simulink model "Linear_Moving_Setpoint_SS_Int"  (R2021b)
settings: Solver=VariableStepAuto  StartTime=tspan(1)  StopTime=tspan(2)  RelTol=1e-9
undefined symbols (not defined in the file): K1, K2, r_sim, x_0
settings Model: Creator=domin  LastModifiedBy=domin
settings SolverCC: AlgebraicLoopSolver=TrustRegion
settings DebuggingCC: SFMachineParentedDataDiag=warning

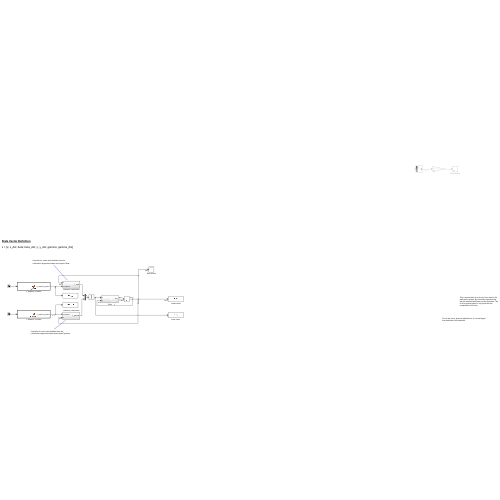
[thumbnail: Simulink's stored preview of the top-level diagram]
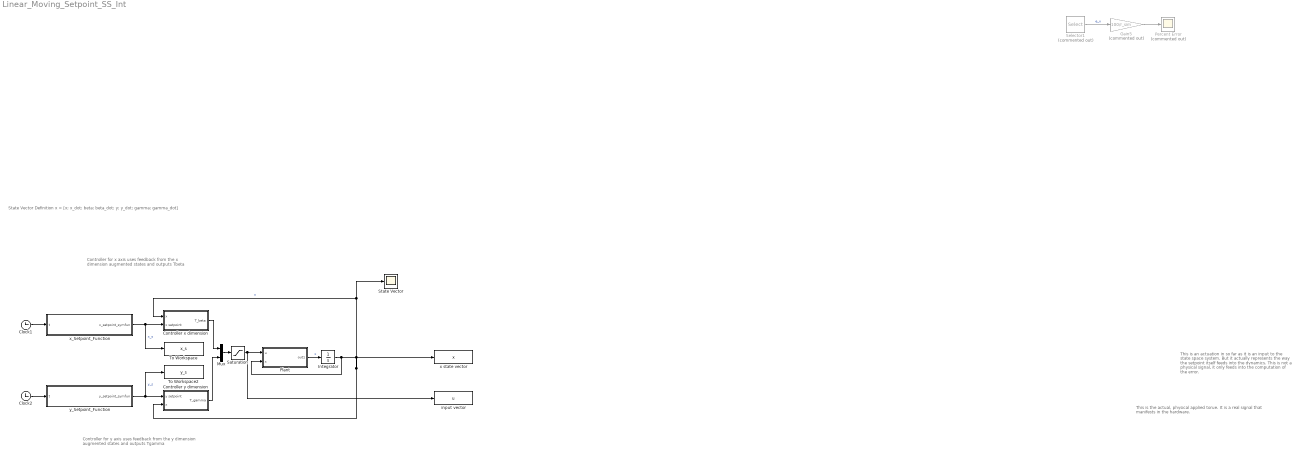
== system Linear_Moving_Setpoint_SS_Int ==
  note: Controller for y axis uses feedback from the
      | y dimension augmented states and outputs Tgamma
  note: State Vector Definition
      |
      | x = [x; x_dot; beta; beta_dot; y; y_dot; gamma; gamma_dot]
  note: This is the actual, physical applied torue. It is a real signal
      | that manifests in the hardware.
  note: This is an actuation in so far as it is an input to the
      | state space system. But it actually represents the
      | way the setpoint itself feeds into the dynamics. This
      | is not a physical signal, it only feeds into the
      | computation of the error.
  note: Controller for x axis uses feedback from the
      | x dimension augmented states and outputs Tbeta
  Clock1 : Clock
  Clock2 : Clock
  Controller x dimension : Subsystem
  Controller y dimension : Subsystem
  Gain5 : Gain  Commented=on  Gain=100/r_sim
  Integrator : Integrator  InitialCondition=x_0
  Mux : Mux  Inputs=2
  Percent Error : Scope  Commented=on
  Plant : Subsystem
  Saturation : Saturate  UpperLimit=73/1000  LowerLimit=-73/1000
  Selector1 : Selector  Commented=on  InputPortWidth=5  IndexOptions=Index vector (dialog)  Indices=[1]  OutputSizes=1
  State Vector : Scope
  To Workspace : ToWorkspace  VariableName=x_s  SampleTime=-1
  To Workspace2 : ToWorkspace  VariableName=y_s  SampleTime=-1
  input vector : ToWorkspace  VariableName=u  SampleTime=-1
  x state vector : ToWorkspace  VariableName=x  SampleTime=-1
  x_Setpoint_Function : MATLAB Function  TreatAsAtomicUnit=on
  y_Setpoint_Function : MATLAB Function  TreatAsAtomicUnit=on
  wires:
  Integrator/1 -> Plant/2(x), x state vector/1, Controller x dimension/1(x), State Vector/1, Controller y dimension/2(x)  "x"
  Plant/1(out1) -> Integrator/1  "x"
  Clock1/1 -> x_Setpoint_Function/1(t)
  Gain5/1 -> Percent Error/1
  Selector1/1 -> Gain5/1  "e_x"
  Clock2/1 -> y_Setpoint_Function/1(t)
  Controller x dimension/1(T_beta) -> Mux/1
  Controller y dimension/1(T_gamma) -> Mux/2
  x_Setpoint_Function/1(x_setpoint_symfun) -> To Workspace/1, Controller x dimension/2(x setpoint)  "x_s"
  y_Setpoint_Function/1(y_setpoint_symfun) -> To Workspace2/1, Controller y dimension/1(y setpoint)  "y_s"
  Mux/1 -> Saturation/1
  Saturation/1 -> Plant/1(u), input vector/1

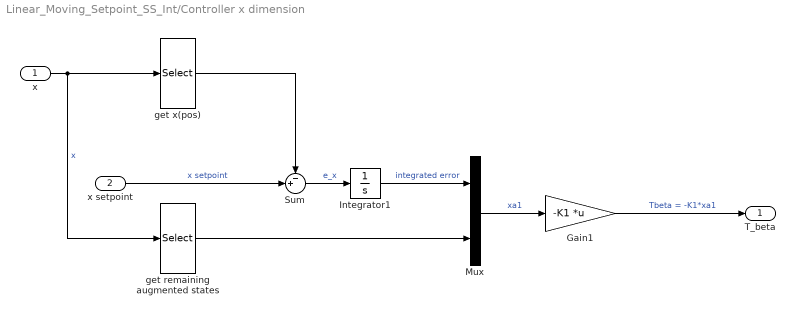
== system Linear_Moving_Setpoint_SS_Int/Controller x dimension ==
  x : Inport
  x setpoint : Inport  Port=2
  Gain1 : Gain  Gain=-K1  Multiplication=Matrix(K*u)
  Integrator1 : Integrator
  Mux : Mux  Inputs=2
  Sum : Sum  Inputs=-+|
  get remaining augmented states : Selector  InputPortWidth=8  IndexOptions=Index vector (dialog)  Indices=[1,2,3,4]  OutputSizes=1
  get x(pos) : Selector  InputPortWidth=8  IndexOptions=Index vector (dialog)  Indices=[1]  OutputSizes=1
  T_beta : Outport
  wires:
  get remaining augmented states/1 -> Mux/2
  Gain1/1 -> T_beta/1  "Tbeta = -K1*xa1"
  get x(pos)/1 -> Sum/1
  Mux/1 -> Gain1/1  "xa1"
  Sum/1 -> Integrator1/1  "e_x"
  Integrator1/1 -> Mux/1  "integrated error"
  x setpoint/1 -> Sum/2  "x setpoint"
  x/1 -> get remaining augmented states/1, get x(pos)/1  "x"

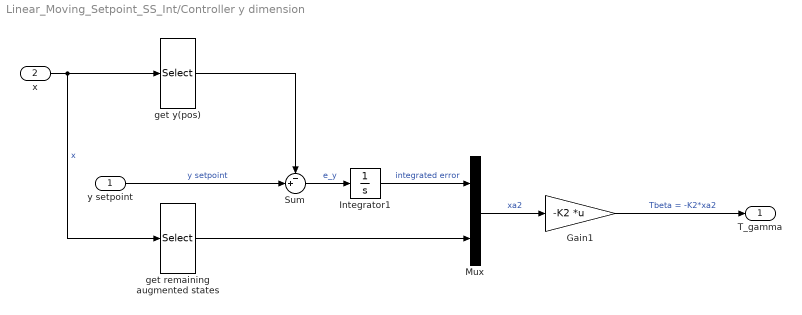
== system Linear_Moving_Setpoint_SS_Int/Controller y dimension ==
  y setpoint : Inport
  x : Inport  Port=2
  Gain1 : Gain  Gain=-K2  Multiplication=Matrix(K*u)
  Integrator1 : Integrator
  Mux : Mux  Inputs=2
  Sum : Sum  Inputs=-+|
  get remaining augmented states : Selector  InputPortWidth=8  IndexOptions=Index vector (dialog)  Indices=[5,6,7,8]  OutputSizes=1
  get y(pos) : Selector  InputPortWidth=8  IndexOptions=Index vector (dialog)  Indices=[2]  OutputSizes=1
  T_gamma : Outport
  wires:
  x/1 -> get y(pos)/1, get remaining augmented states/1  "x"
  y setpoint/1 -> Sum/2  "y setpoint"
  Integrator1/1 -> Mux/1  "integrated error"
  Sum/1 -> Integrator1/1  "e_y"
  Mux/1 -> Gain1/1  "xa2"
  get y(pos)/1 -> Sum/1
  Gain1/1 -> T_gamma/1  "Tbeta = -K2*xa2"
  get remaining augmented states/1 -> Mux/2

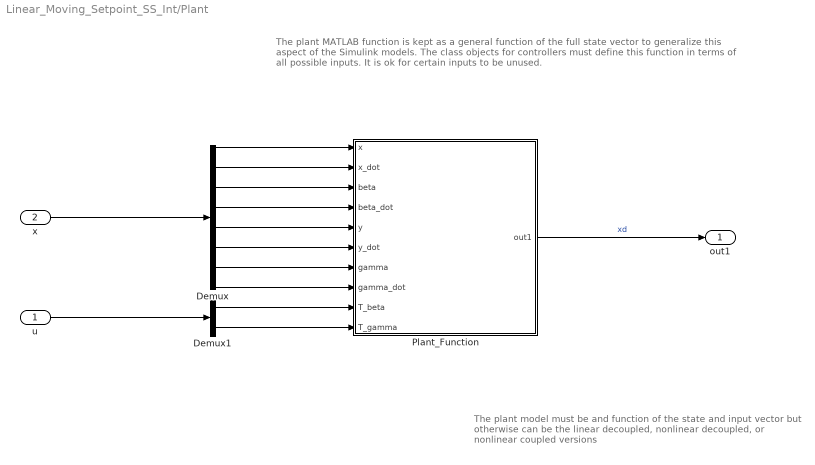
== system Linear_Moving_Setpoint_SS_Int/Plant ==
  note: The plant model must be and function of the state and input vector
      |  but otherwise can be the linear decoupled, nonlinear decoupled,
      | or nonlinear coupled versions
  note: The plant MATLAB function is kept as a general function of the full state vector
      | to generalize this aspect of the Simulink models. The class objects for controllers must define this function in terms of all possible inputs. It is ok for certain inputs to be unused.
  u : Inport
  x : Inport  Port=2
  Demux : Demux  Outputs=8
  Demux1 : Demux  Outputs=2
  Plant_Function : MATLAB Function  TreatAsAtomicUnit=on
  out1 : Outport
  wires:
  Demux/1 -> Plant_Function/1(x)
  x/1 -> Demux/1
  Plant_Function/1(out1) -> out1/1  "xd"
  Demux/2 -> Plant_Function/2(x_dot)
  Demux/4 -> Plant_Function/4(beta_dot)
  Demux/3 -> Plant_Function/3(beta)
  Demux/6 -> Plant_Function/6(y_dot)
  Demux/5 -> Plant_Function/5(y)
  Demux1/2 -> Plant_Function/10(T_gamma)
  u/1 -> Demux1/1
  Demux/8 -> Plant_Function/8(gamma_dot)
  Demux1/1 -> Plant_Function/9(T_beta)
  Demux/7 -> Plant_Function/7(gamma)

== matlab function Linear_Moving_Setpoint_SS_Int/Plant/Plant_Function ==
  data: x input; out1 output; x_dot input; beta input; beta_dot input; y input; y_dot input; gamma input; gamma_dot input; T_beta input; T_gamma input
function out1 = xdot(x,x_dot,beta,beta_dot,y,y_dot,gamma,gamma_dot,T_beta,T_gamma)
%#codegen

%    This function was generated by the Symbolic Math Toolbox version 9.0.
%    04-Nov-2021 01:00:01

mt1 = [x_dot,T_beta.*(-1.772680446266138e+1)+beta.*4.011095116498257-x.*5.216998553361243,beta_dot,T_beta.*3.835784582337856e+2+beta.*6.482947197685378e+1+x.*1.128871402582031e+2,y_dot,T_gamma.*1.772680446266138e+1-gamma.*4.011095116498257-y.*5.216998553361243,gamma_dot];
mt2 = [T_gamma.*3.835784582337856e+2+gamma.*6.482947197685378e+1-y.*1.128871402582031e+2];
out1 = reshape([mt1,mt2],8,1);

== matlab function Linear_Moving_Setpoint_SS_Int/x_Setpoint_Function ==
  data: t input; x_setpoint_symfun output
function x_setpoint_symfun = x_setpoint(t)
%#codegen

%    This function was generated by the Symbolic Math Toolbox version 9.0.
%    04-Nov-2021 01:00:01

x_setpoint_symfun = sin(t.*pi.*(2.0./3.0))./1.0e+1;

== matlab function Linear_Moving_Setpoint_SS_Int/y_Setpoint_Function ==
  data: t input; y_setpoint_symfun output
function y_setpoint_symfun = y_setpoint(t)
%#codegen

%    This function was generated by the Symbolic Math Toolbox version 9.0.
%    04-Nov-2021 01:00:01

y_setpoint_symfun = sin(pi./2.0+t.*pi.*(2.0./3.0))./1.0e+1;
